simulink model "sfun_size_test"  (R2017a)
settings: Solver=VariableStepAuto  StartTime=0.0  StopTime=10.0  RelTol=1e-3
libraries: simulink x1
settings Model: Creator=eruffaldi  LastModifiedBy=eruffaldi

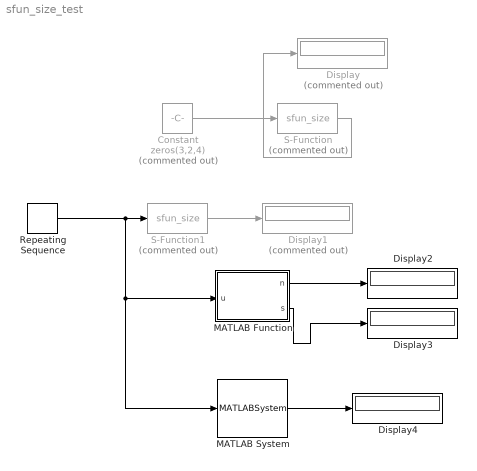
== system sfun_size_test ==
  Constant : Constant  Commented=on  Value=zeros(3,2,4)
  Display : Display  Commented=on
  Display1 : Display  Commented=on
  Display2 : Display
  Display3 : Display
  Display4 : Display
  MATLAB Function : MATLAB Function  TreatAsAtomicUnit=on
  MATLAB System : MATLABSystem  System=sfun_size_sys  SimulateUsing=Code generation
      mask Type: sfun_size_sys
      mask Display:
      | disp('sfun_size_sys');
      | port_label('input',1,'u');
      | port_label('output',1,'y');
  Repeating Sequence : simulink/Sources/Repeating Sequence  rep_seq_t=[0 2]  rep_seq_y=[0 2]
  S-Function : S-Function  Commented=on  FunctionName=sfun_size  SFunctionDeploymentMode=off  EnableBusSupport=off
  S-Function1 : S-Function  Commented=on  FunctionName=sfun_size  SFunctionDeploymentMode=off  EnableBusSupport=off
  wires:
  Constant/1 -> S-Function/1
  S-Function/1 -> Display/1
  S-Function1/1 -> Display1/1
  Repeating Sequence/1 -> MATLAB System/1, MATLAB Function/1(u), S-Function1/1
  MATLAB Function/1(n) -> Display2/1
  MATLAB Function/2(s) -> Display3/1
  MATLAB System/1 -> Display4/1

== matlab function sfun_size_test/MATLAB Function ==
  data: u input; n output; s output
function [n,s] = fcn(u)

n = ndims(u);
s = [size(u,1) size(u,2) size(u,3) size(u,4)];
